simulink library "SixDoF_Lib"  (R2016b)
settings: Solver=VariableStepAuto  StartTime=0.0  StopTime=10.0  RelTol=1e-3
undefined symbols (not defined in the file): AC, TrimCondition
libraries: OpenFlightUtilLib x3
settings Model: Creator=UAVLAB  LastModifiedBy=UAVLAB

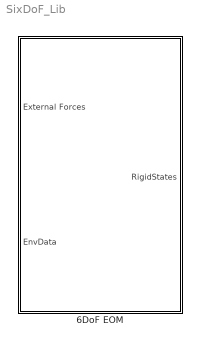
== system SixDoF_Lib ==
  6DoF EOM : Subsystem  mask(6DoF EoM (Body Axis)){units=Metric (MKS), mtype=Fixed, rep=Euler Angles, xme_0=TrimCondition.InertialIni, Vm_0=TrimCondition.VelocitiesIni, eul_0=TrimCondition.AttitudeIni, pm_0=TrimCondition.RatesIni, mass_0=AC.MassP.mass_kg, mass_e=0.5, mass_f=2.0, inertia=AC.MassP.I_B_kgm2, inertia_e=eye(3), inertia_f=2*eye(3), k_quat=1.0}
      mask prompts: mtype "Mass type:"; rep "Representation:"; xme_0 "Initial position in inertial axes [Xe,Ye,Ze]:"; Vm_0 "Initial velocity in body axes [U,v,w]:"; eul_0 "Initial Euler orientation [roll, pitch, yaw]:"; pm_0 "Initial body rotation rates [p,q,r]:"; mass_0 "Initial mass:"; mass_e "Empty mass:"; mass_f "Full mass:"; inertia_e "Empty inertia matrix:"; inertia_f "Full inertia matrix:"; k_quat "Gain for quaternion normalization:"
      mask help:
      | Integrate the six-degrees-of-freedom equations of motion in body axis.
      |
      | This block has been modified from the original Aerospace Blockset
      | implementation. The inertial position vector (Xe) is no longer computed.
      | The original block did not have a way to add steady state winds to the
      | inertial velocities (Ve) prior to integrating to get Xe. Therefore, this
      | step is performed in the Auxiliary Equations block.
      mask Help: eval('asbhelp(''sixdof_euler_angles'')');
      mask TypeOptions units: Metric (MKS) | English (Velocity in ft/s) | English (Velocity in kts)
      mask TypeOptions mtype: Fixed | Simple Variable | Custom Variable
      mask Callback mtype: aeroicon('aeroblk6dofbody');
      mask TypeOptions rep: Euler Angles | Quaternion
      mask Callback rep: aeroicon('aeroblk6dofbody');

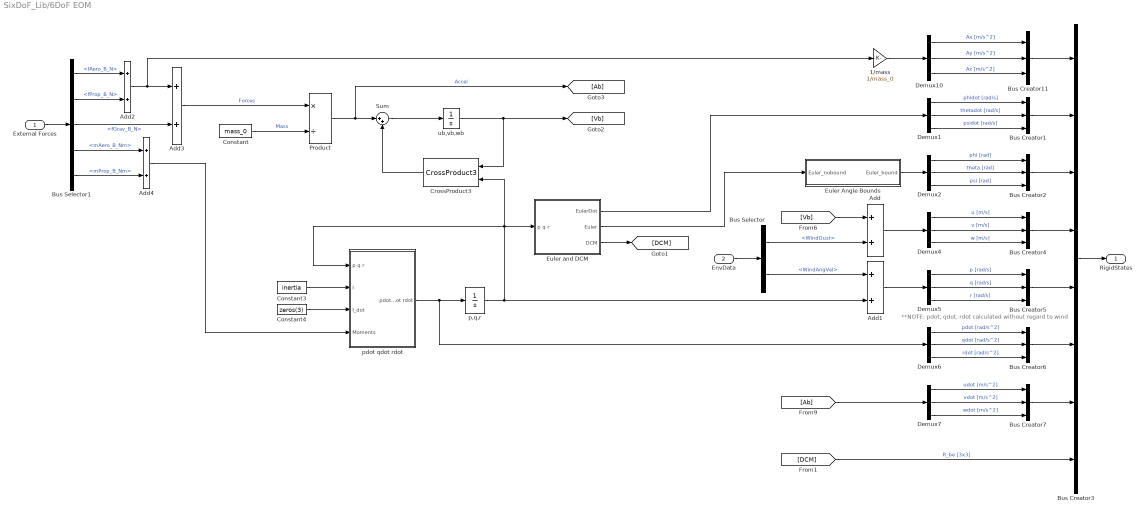
== system SixDoF_Lib/6DoF EOM ==
  note: **NOTE: pdot, qdot, rdot calculated without regard to wind
  External Forces : Inport
  EnvData : Inport  Port=2  OutDataTypeStr=Bus: EnvData
  1/mass : Gain  Gain=1/mass_0
  Add{,1..4} (5 alike) : Sum
  Bus Creator{1..2,4..7,11} (7 alike) : BusCreator  Inputs=3
  Bus Selector : BusSelector  OutputSignals=WindGust,WindAngVel
  Bus Selector1 : BusSelector  OutputSignals=fAero_B_N,fProp_B_N,fGrav_B_N,mAero_B_Nm,mProp_B_Nm
  Bus Creator3 : BusCreator  Inputs=8  OutDataTypeStr=Bus: RigidStates
      settings: InheritFromInputs=off
  Constant : Constant  Value=mass_0  OutDataTypeStr=Inherit: Inherit via back propagation
  Constant3 : Constant  Value=inertia  OutDataTypeStr=Inherit: Inherit via back propagation
  Constant4 : Constant  Value=zeros(3)
  CrossProduct3 : OpenFlightUtilLib/Math/CrossProduct3
  Demux{1..2,4..7,10} (7 alike) : Demux  Outputs=3
  Euler Angle Bounds : Subsystem
  Euler and DCM : Subsystem
  Product : Product  Inputs=*/  SaturateOnIntegerOverflow=on  OutDataTypeStr=Inherit: Same as first input
  Sum : Sum  Inputs=|++  SaturateOnIntegerOverflow=on
  "p,q,r " : Integrator  InitialCondition=pm_0
  pdot qdot rdot : Subsystem
  ub,vb,wb : Integrator  InitialCondition=convvel(Vm_0,'m/s','m/s')
  RigidStates : Outport  OutDataTypeStr=Bus: RigidStates
  wires:
  [DCM] -> Bus Creator3/8  "R_be [3x3]"
  Bus Creator11/1 -> Bus Creator3/1
  Bus Creator2/1 -> Bus Creator3/3
  Bus Creator1/1 -> Bus Creator3/2
  Bus Creator7/1 -> Bus Creator3/7
  Bus Creator6/1 -> Bus Creator3/6
  Bus Creator5/1 -> Bus Creator3/5
  Bus Creator4/1 -> Bus Creator3/4
  Bus Creator3/1 -> RigidStates/1
  Add4/1 -> pdot qdot rdot/4(Moments)
  Bus Selector1/5 -> Add4/2  "<mProp_B_Nm>"
  Bus Selector1/4 -> Add4/1  "<mAero_B_Nm>"
  Bus Selector1/3 -> Add3/2  "<fGrav_B_N>"
  Bus Selector1/2 -> Add2/2  "<fProp_B_N>"
  Bus Selector1/1 -> Add2/1  "<fAero_B_N>"
  External Forces/1 -> Bus Selector1/1
  Demux10/3 -> Bus Creator11/3  "Az [m/s^2]"
  Demux10/2 -> Bus Creator11/2  "Ay [m/s^2]"
  Demux10/1 -> Bus Creator11/1  "Ax [m/s^2]"
  1/mass/1 -> Demux10/1
  Add2/1 -> 1/mass/1, Add3/1
  Euler Angle Bounds/1(Euler_bound) -> Demux2/1
  Demux2/1 -> Bus Creator2/1  "phi [rad]"
  Demux2/2 -> Bus Creator2/2  "theta [rad]"
  Demux2/3 -> Bus Creator2/3  "psi [rad]"
  Euler and DCM/2(Euler) -> Euler Angle Bounds/1(Euler_nobound)
  Euler and DCM/1(EulerDot) -> Demux1/1
  Demux1/1 -> Bus Creator1/1  "phidot [rad/s]"
  Demux1/2 -> Bus Creator1/2  "thetadot [rad/s]"
  Demux1/3 -> Bus Creator1/3  "psidot [rad/s]"
  Demux7/1 -> Bus Creator7/1  "udot [m/s^2]"
  Demux7/2 -> Bus Creator7/2  "vdot [m/s^2]"
  Demux7/3 -> Bus Creator7/3  "wdot [m/s^2]"
  [Ab] -> Demux7/1
  Demux6/1 -> Bus Creator6/1  "pdot [rad/s^2]"
  Demux6/2 -> Bus Creator6/2  "qdot [rad/s^2]"
  Demux6/3 -> Bus Creator6/3  "rdot [rad/s^2]"
  pdot qdot rdot/1(pdot qdot rdot) -> "p,q,r "/1, Demux6/1
  Add1/1 -> Demux5/1
  Demux5/1 -> Bus Creator5/1  "p [rad/s]"
  Demux5/2 -> Bus Creator5/2  "q [rad/s]"
  Demux5/3 -> Bus Creator5/3  "r [rad/s]"
  "p,q,r "/1 -> Add1/2, Euler and DCM/1("p q r "), CrossProduct3/2, pdot qdot rdot/1(p q r)
  Demux4/1 -> Bus Creator4/1  "u [m/s]"
  Demux4/2 -> Bus Creator4/2  "v [m/s]"
  Demux4/3 -> Bus Creator4/3  "w [m/s]"
  Add/1 -> Demux4/1
  [Vb] -> Add/1
  Bus Selector/2 -> Add1/1  "<WindAngVel>"
  Bus Selector/1 -> Add/2  "<WindGust>"
  EnvData/1 -> Bus Selector/1
  CrossProduct3/1 -> Sum/2
  Sum/1 -> ub,vb,wb/1
  Product/1 -> [Ab], Sum/1  "Accel"
  Euler and DCM/3(DCM) -> [DCM]
  Constant/1 -> Product/2  "Mass"
  Add3/1 -> Product/1  "Forces"
  ub,vb,wb/1 -> [Vb], CrossProduct3/1
  Constant4/1 -> pdot qdot rdot/3(I_dot)
  Constant3/1 -> pdot qdot rdot/2(I)

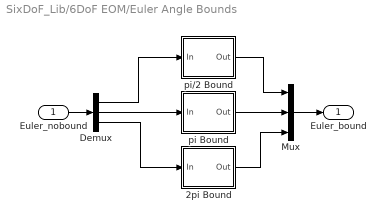
== system SixDoF_Lib/6DoF EOM/Euler Angle Bounds ==
  Euler_nobound : Inport
  2pi Bound : Subsystem
  Demux : Demux  Outputs=3
  Mux : Mux  Inputs=3
  pi Bound : Subsystem
  pi/2 Bound : Subsystem
  Euler_bound : Outport
  wires:
  pi Bound/1(Out) -> Mux/2
  pi/2 Bound/1(Out) -> Mux/1
  Mux/1 -> Euler_bound/1
  Euler_nobound/1 -> Demux/1
  Demux/1 -> pi/2 Bound/1(In)
  Demux/2 -> pi Bound/1(In)
  Demux/3 -> 2pi Bound/1(In)
  2pi Bound/1(Out) -> Mux/3

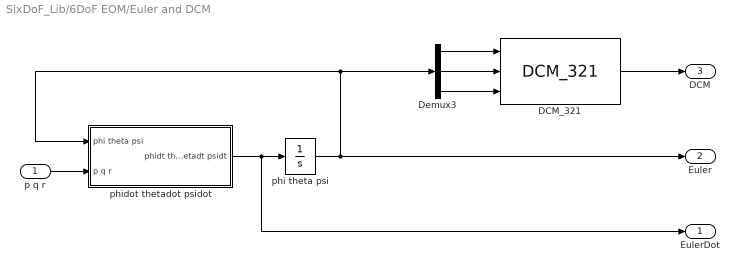
== system SixDoF_Lib/6DoF EOM/Euler and DCM ==
  "p q r " : Inport
  DCM_321 : OpenFlightUtilLib/Transformations/DCM_321
  Demux3 : Demux  Outputs=3
  phi theta psi : Integrator  InitialCondition=eul_0
  phidot thetadot psidot : Subsystem
  EulerDot : Outport
  Euler : Outport  Port=2
  DCM : Outport  Port=3
  wires:
  phi theta psi/1 -> phidot thetadot psidot/1(phi theta psi), Demux3/1, Euler/1
  phidot thetadot psidot/1(phidt thetadt psidt) -> EulerDot/1, phi theta psi/1
  "p q r "/1 -> phidot thetadot psidot/2(p q r)
  DCM_321/1 -> DCM/1
  Demux3/3 -> DCM_321/3
  Demux3/2 -> DCM_321/2
  Demux3/1 -> DCM_321/1

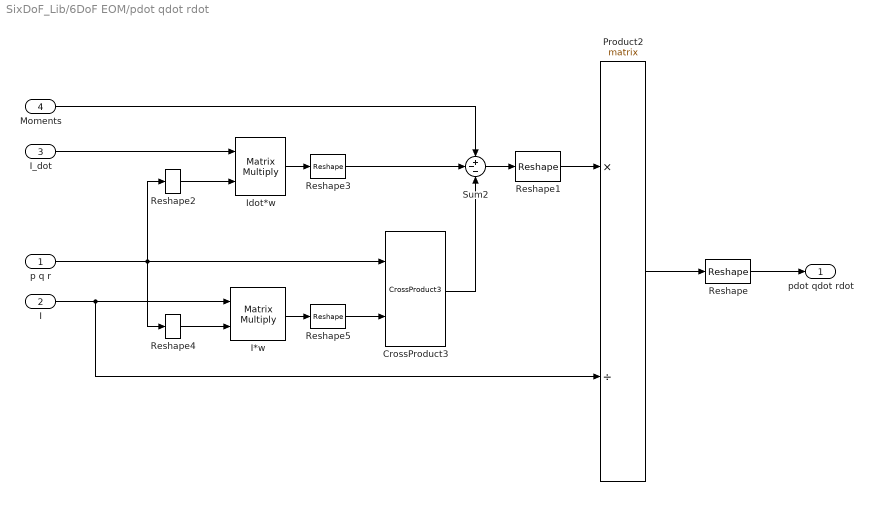
== system SixDoF_Lib/6DoF EOM/pdot qdot rdot ==
  p q r : Inport
  I : Inport  Port=2
  I_dot : Inport  Port=3
  Moments : Inport  Port=4
  CrossProduct3 : OpenFlightUtilLib/Math/CrossProduct3
  I*w : Product  Multiplication=Matrix(*)  SaturateOnIntegerOverflow=on  InputSameDT=on  OutDataTypeStr=Inherit: Same as first input
  Idot*w : Product  Multiplication=Matrix(*)  SaturateOnIntegerOverflow=on  InputSameDT=on  OutDataTypeStr=Inherit: Same as first input
  Product2 : Product  Inputs=*/  Multiplication=Matrix(*)  SaturateOnIntegerOverflow=on  OutDataTypeStr=Inherit: Same as first input
  Reshape : Reshape
  Reshape1 : Reshape  OutputDimensionality=Row vector (2-D)
  Reshape2 : Reshape  OutputDimensionality=Column vector (2-D)
  Reshape3 : Reshape
  Reshape4 : Reshape  OutputDimensionality=Column vector (2-D)
  Reshape5 : Reshape
  Sum2 : Sum  Inputs=+--  SaturateOnIntegerOverflow=on
  pdot qdot rdot : Outport
  wires:
  Reshape1/1 -> Product2/1
  Reshape5/1 -> CrossProduct3/2
  CrossProduct3/1 -> Sum2/3
  Reshape3/1 -> Sum2/2
  Moments/1 -> Sum2/1
  Sum2/1 -> Reshape1/1
  Product2/1 -> Reshape/1
  p q r/1 -> Reshape2/1, Reshape4/1, CrossProduct3/1
  Reshape/1 -> pdot qdot rdot/1
  Reshape2/1 -> Idot*w/2
  Idot*w/1 -> Reshape3/1
  I_dot/1 -> Idot*w/1
  Reshape4/1 -> I*w/2
  I/1 -> Product2/2, I*w/1
  I*w/1 -> Reshape5/1

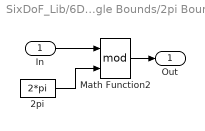
== system SixDoF_Lib/6DoF EOM/Euler Angle Bounds/2pi Bound ==
  In : Inport
  2pi : Constant  Value=2*pi
  Math Function2 : Math  Operator=mod  SaturateOnIntegerOverflow=on
  Out : Outport
  wires:
  Math Function2/1 -> Out/1
  2pi/1 -> Math Function2/2
  In/1 -> Math Function2/1

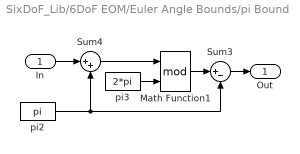
== system SixDoF_Lib/6DoF EOM/Euler Angle Bounds/pi Bound ==
  In : Inport
  Math Function1 : Math  Operator=mod  SaturateOnIntegerOverflow=on
  Sum3 : Sum  Inputs=|+-  SaturateOnIntegerOverflow=on  InputSameDT=on  OutDataTypeStr=Inherit: Same as first input
  Sum4 : Sum  Inputs=|++  SaturateOnIntegerOverflow=on  InputSameDT=on  OutDataTypeStr=Inherit: Same as first input
  pi2 : Constant  Value=pi
  pi3 : Constant  Value=2*pi
  Out : Outport
  wires:
  Math Function1/1 -> Sum3/1
  pi3/1 -> Math Function1/2
  In/1 -> Sum4/1
  Sum4/1 -> Math Function1/1
  pi2/1 -> Sum4/2, Sum3/2
  Sum3/1 -> Out/1

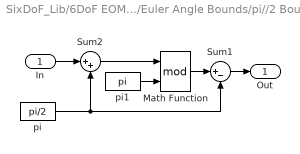
== system SixDoF_Lib/6DoF EOM/Euler Angle Bounds/pi//2 Bound ==
  In : Inport
  Math Function : Math  Operator=mod  SaturateOnIntegerOverflow=on
  Sum1 : Sum  Inputs=|+-  SaturateOnIntegerOverflow=on  InputSameDT=on  OutDataTypeStr=Inherit: Same as first input
  Sum2 : Sum  Inputs=|++  SaturateOnIntegerOverflow=on  InputSameDT=on  OutDataTypeStr=Inherit: Same as first input
  pi : Constant  Value=pi/2
  pi1 : Constant  Value=pi
  Out : Outport
  wires:
  Sum1/1 -> Out/1
  pi/1 -> Sum1/2, Sum2/2
  Sum2/1 -> Math Function/1
  In/1 -> Sum2/1
  pi1/1 -> Math Function/2
  Math Function/1 -> Sum1/1

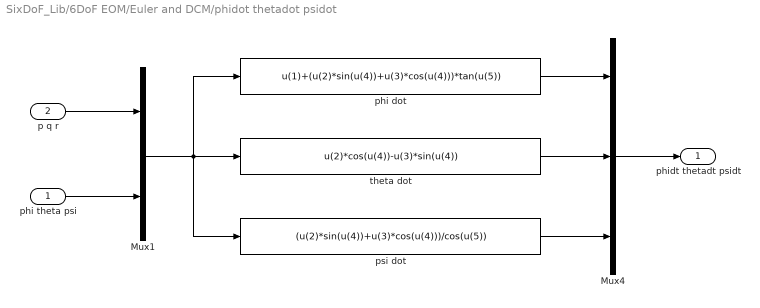
== system SixDoF_Lib/6DoF EOM/Euler and DCM/phidot thetadot psidot ==
  phi theta psi : Inport
  p q r : Inport  Port=2
  Mux1 : Mux  Inputs=[3 3]
  Mux4 : Mux  Inputs=3
  phi dot : Fcn  Expr=u(1)+(u(2)*sin(u(4))+u(3)*cos(u(4)))*tan(u(5))
  psi dot : Fcn  Expr=(u(2)*sin(u(4))+u(3)*cos(u(4)))/cos(u(5))
  theta dot : Fcn  Expr=u(2)*cos(u(4))-u(3)*sin(u(4))
  phidt thetadt psidt : Outport  InitialOutput=0
  wires:
  phi theta psi/1 -> Mux1/2
  Mux4/1 -> phidt thetadt psidt/1
  Mux1/1 -> psi dot/1, theta dot/1, phi dot/1
  phi dot/1 -> Mux4/1
  theta dot/1 -> Mux4/2
  psi dot/1 -> Mux4/3
  p q r/1 -> Mux1/1
